simulink model "SwtsLPV"  (Simulink 7.4)
settings: Solver=FixedStepDiscrete  StartTime=0.0  StopTime=100.0  FixedStep=h  RelTol=1e-3
values from neighbouring files (symbols this model uses):
  h = 0.1    [ex04_lti_wts.m]    (also in ex05_lti_wts_batch.m; ex07_lti_wts_mcs.m; ex08_lti_wts_bootstrap.m; ex17_c2d_f16.m = linspace(5000,25000,length(t))')
  M = linspace(0.4,0.6,length(t))'    [ex17_c2d_f16.m]    (also in ex19_lpv_flap.m = idafflpv(A12,B12,C12,D12,eye(2),zeros(2,1),1); ex19b_lpv_stable_predictor.m = idafflpv(A12,B12,C12,D12,eye(2),zeros(2,1),1); ex19c_lpv_sparse.m = idafflpv(A12,B12,C12,D12,eye(2),zeros(2,1),1); ex20_lpv_mimo.m = idafflpv(Alpv,Blpv,Clpv,Dlpv,Klpv,[],1))
libraries: simulink x1
settings Model: Creator=ihoutzager  LastModifiedBy=ivohoutzager
settings OptimizationCC: InitFltsAndDblsToZero=on
settings DebuggingCC: SaveWithParameterizedLinksMsg=none  SignalResolutionControl=TryResolveAllWithWarning
settings GRTTargetCC: TargetFcnLib=ansi_tfl_tmw.mat

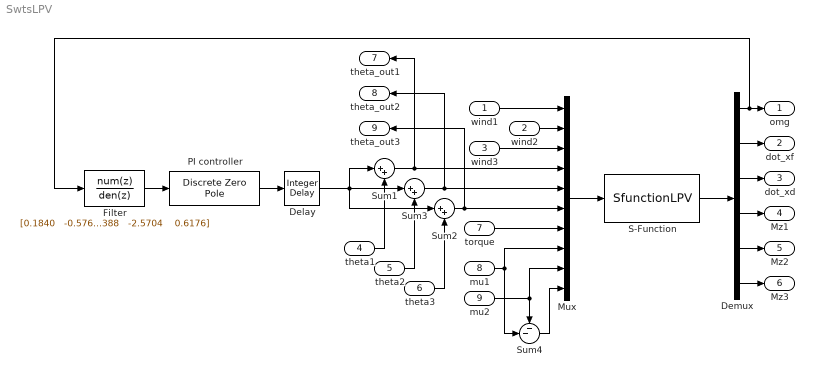
== system SwtsLPV ==
  wind1 : Inport  OutDataType=sfix(16)  OutScaling=2^0
  wind2 : Inport  Port=2  OutDataType=sfix(16)  OutScaling=2^0
  wind3 : Inport  Port=3  OutDataType=sfix(16)  OutScaling=2^0
  theta1 : Inport  Port=4  OutDataType=sfix(16)  OutScaling=2^0
  theta2 : Inport  Port=5  OutDataType=sfix(16)  OutScaling=2^0
  theta3 : Inport  Port=6  OutDataType=sfix(16)  OutScaling=2^0
  torque : Inport  Port=7  OutDataType=sfix(16)  OutScaling=2^0
  mu1 : Inport  Port=8  OutDataType=sfix(16)  OutScaling=2^0
  mu2 : Inport  Port=9  OutDataType=sfix(16)  OutScaling=2^0
  Delay : simulink/Discrete/Integer Delay  vinit=0.0  samptime=h  NumDelays=1
  Demux : Demux  Outputs=6
  Filter : DiscreteTransferFcn  Numerator="[0.1840   -0.5760    0.8115   -0.5760    0.1840]"  Denominator="[1.0000   -3.2569    4.2388   -2.5704    0.6176]"  SampleTime=0.1
  Mux : Mux  Inputs=10
  PI controller : DiscreteZeroPole  Zeros=[0.99]  Poles=[1]  Gain=46.9335  SampleTime=h
  S-Function : S-Function  FunctionName=SfunctionLPV  Parameters=M.a,M.b,M.c,M.d  EnableBusSupport=off
  Sum1 : Sum  Inputs=|++  OutDataType=sfix(16)  OutScaling=2^0
  Sum2 : Sum  Inputs=|++  OutDataType=sfix(16)  OutScaling=2^0
  Sum3 : Sum  Inputs=|++  OutDataType=sfix(16)  OutScaling=2^0
  Sum4 : Sum  Inputs=--|  OutDataType=sfix(16)  OutScaling=2^0
  omg : Outport  SampleTime=h  OutDataType=sfix(16)  OutScaling=2^0
  dot_xf : Outport  Port=2  SampleTime=h  OutDataType=sfix(16)  OutScaling=2^0
  dot_xd : Outport  Port=3  SampleTime=h  OutDataType=sfix(16)  OutScaling=2^0
  Mz1 : Outport  Port=4  SampleTime=h  OutDataType=sfix(16)  OutScaling=2^0
  Mz2 : Outport  Port=5  SampleTime=h  OutDataType=sfix(16)  OutScaling=2^0
  Mz3 : Outport  Port=6  SampleTime=h  OutDataType=sfix(16)  OutScaling=2^0
  theta_out1 : Outport  Port=7  SampleTime=h  OutDataType=sfix(16)  OutScaling=2^0
  theta_out2 : Outport  Port=8  SampleTime=h  OutDataType=sfix(16)  OutScaling=2^0
  theta_out3 : Outport  Port=9  SampleTime=h  OutDataType=sfix(16)  OutScaling=2^0
  wires:
  S-Function/1 -> Demux/1
  Mux/1 -> S-Function/1
  mu1/1 -> Mux/8, Sum4/2
  mu2/1 -> Mux/9, Sum4/1
  wind3/1 -> Mux/3
  wind1/1 -> Mux/1
  wind2/1 -> Mux/2
  Sum4/1 -> Mux/10
  Delay/1 -> Sum2/1, Sum3/1, Sum1/1
  Demux/6 -> Mz3/1
  Demux/5 -> Mz2/1
  Demux/4 -> Mz1/1
  Demux/3 -> dot_xd/1
  Demux/2 -> dot_xf/1
  Demux/1 -> omg/1, Filter/1
  Sum2/1 -> Mux/6, theta_out3/1
  Sum3/1 -> Mux/5, theta_out2/1
  Sum1/1 -> Mux/4, theta_out1/1
  theta1/1 -> Sum1/2
  theta2/1 -> Sum3/2
  theta3/1 -> Sum2/2
  torque/1 -> Mux/7
  PI controller/1 -> Delay/1
  Filter/1 -> PI controller/1
